simulink model "SCM_PD_PENDULUM_OKE"  (R2017b)
settings: Solver=FixedStepAuto  StartTime=0.0  StopTime=40  FixedStep=0.01  RelTol=1e-3
settings Model: Creator=DELL  LastModifiedBy=DELL

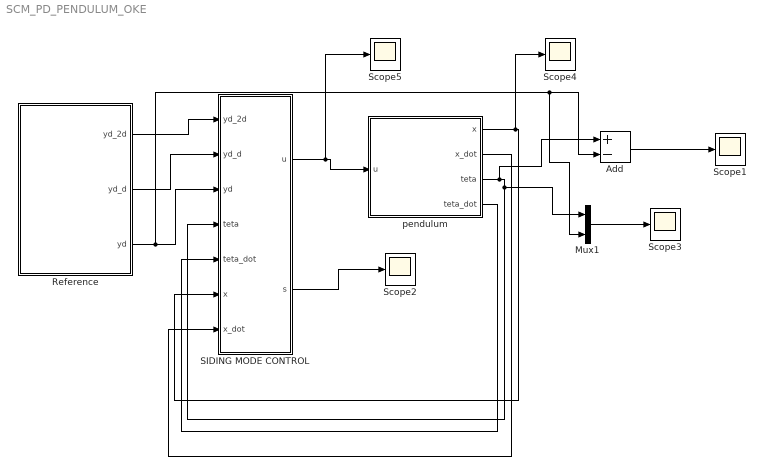
== system SCM_PD_PENDULUM_OKE ==
  Add : Sum  Inputs=+-
  Mux1 : Mux  Inputs=2
  Reference : Subsystem
  "SIDING MODE CONTROL " : MATLAB Function  TreatAsAtomicUnit=on
  Scope{1..5} (5 alike) : Scope
  pendulum : Subsystem
  wires:
  Add/1 -> Scope1/1
  Reference/1(yd_2d) -> "SIDING MODE CONTROL "/1(yd_2d)
  Reference/2(yd_d) -> "SIDING MODE CONTROL "/2(yd_d)
  Reference/3(yd) -> Mux1/2, Add/2, "SIDING MODE CONTROL "/3(yd)
  pendulum/3(teta) -> Add/1, Mux1/1, "SIDING MODE CONTROL "/4(teta)
  pendulum/4(teta_dot) -> "SIDING MODE CONTROL "/5(teta_dot)
  pendulum/1(x) -> Scope4/1, "SIDING MODE CONTROL "/6(x)
  pendulum/2(x_dot) -> "SIDING MODE CONTROL "/7(x_dot)
  Mux1/1 -> Scope3/1
  "SIDING MODE CONTROL "/1(u) -> Scope5/1, pendulum/1(u)
  "SIDING MODE CONTROL "/2(s) -> Scope2/1

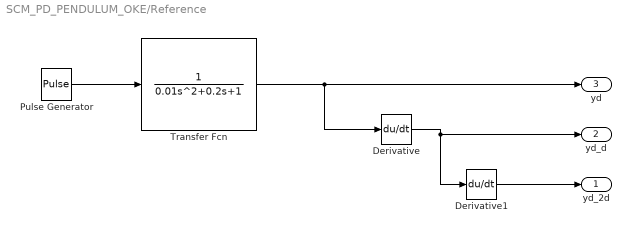
== system SCM_PD_PENDULUM_OKE/Reference ==
  Derivative : Derivative
  Derivative1 : Derivative
  Pulse Generator : DiscretePulseGenerator  PulseType=Time based  Amplitude=pi/3  Period=20  PulseWidth=50
  Transfer Fcn : TransferFcn  Denominator=[0.01 0.2 1]
  yd_2d : Outport  VectorParamsAs1DForOutWhenUnconnected=on
  yd_d : Outport  Port=2  VectorParamsAs1DForOutWhenUnconnected=on
  yd : Outport  Port=3  VectorParamsAs1DForOutWhenUnconnected=on
  wires:
  Transfer Fcn/1 -> Derivative/1, yd/1
  Pulse Generator/1 -> Transfer Fcn/1
  Derivative/1 -> Derivative1/1, yd_d/1
  Derivative1/1 -> yd_2d/1

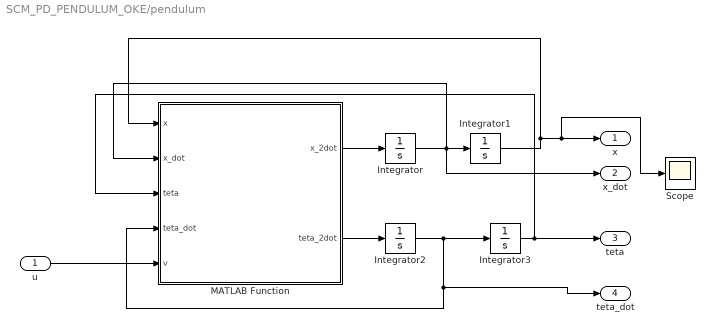
== system SCM_PD_PENDULUM_OKE/pendulum ==
  u : Inport
  Integrator : Integrator
  Integrator1 : Integrator  InitialCondition=0.05
  Integrator2 : Integrator
  Integrator3 : Integrator  InitialCondition=0.05
  MATLAB Function : MATLAB Function  TreatAsAtomicUnit=on
  Scope : Scope
  x : Outport
  x_dot : Outport  Port=2
  teta : Outport  Port=3
  teta_dot : Outport  Port=4
  wires:
  Integrator2/1 -> teta_dot/1, MATLAB Function/4(teta_dot), Integrator3/1
  MATLAB Function/2(teta_2dot) -> Integrator2/1
  Integrator1/1 -> x/1, Scope/1, MATLAB Function/1(x)
  MATLAB Function/1(x_2dot) -> Integrator/1
  Integrator3/1 -> teta/1, MATLAB Function/3(teta)
  Integrator/1 -> x_dot/1, MATLAB Function/2(x_dot), Integrator1/1
  u/1 -> MATLAB Function/5(v)

== matlab function SCM_PD_PENDULUM_OKE/pendulum/MATLAB Function ==
  data: x input; x_2dot output; x_dot input; teta input; teta_dot input; v input; teta_2dot output
function [x_2dot,teta_2dot] = fcn(x,x_dot,teta,teta_dot,v)
global v1 v2
g=9.81; %Gravity(m/s^2)
r=0.051; %Radius of wheel(m)
Mw=0.03; %Mass of wheel(kg)
Mp=1.13; %Mass of body(kg)
Iw=0.000039; %Inertia of the wheel(kg*m^2)
Ip=0.0041; %Inertia of the body(kg*m^2)
L=0.07; %Length to the body's center of mass(m)

%Motor's variables
Km=0.006123; %Motor torque constant(Nm/A)
Ke=0.006087; %Back EMF constant(Vs/rad)
R=3; %Nominal terminal resistance(Ohm)
a1=Mp*L/(Ip+Mp*L^2);
a2=Km*Ke/(R*r*(Ip+Mp*L^2));
a3=Km/(R*(Ip+Mp*L^2));
a4=Mp*g*L/(Ip+Mp*L^2);
b1=2*Km/(R*r*(2*Mw+2*(Iw/r^2)+Mp));
b2=2*Km*Ke/(R*r^2*(2*Mw+2*(Iw/r^2)+Mp));
b3=Mp*L/(2*Mw+2*(Iw/r^2)+Mp);
K=1.0e+03 *[-0.0316   -0.0361    1.6415    0.1272];


teta_2dot = -(a4*teta - 2*a3*v + 2*a2*x + a1*b1*v - a1*b2*x_dot)/(a1*b3 - 1);
x_2dot=-(b1*v - b2*x_dot + a4*b3*teta - 2*a3*b3*v + 2*a2*b3*x)/(a1*b3 - 1);

== matlab function SCM_PD_PENDULUM_OKE/SIDING MODE CONTROL  ==
  data: yd_2d input; u output; yd_d input; yd input; teta input; teta_dot input; s output; x input; x_dot input
function [u,s]= SMC(yd_2d,yd_d,yd,teta,teta_dot,x,x_dot)

g=9.81; %Gravity(m/s^2)
r=0.051; %Radius of wheel(m)
Mw=0.03; %Mass of wheel(kg)
Mp=1.13; %Mass of body(kg)
Iw=0.000039; %Inertia of the wheel(kg*m^2)
Ip=0.0041; %Inertia of the body(kg*m^2)
L=0.07; %Length to the body's center of mass(m)

%Motor's variables
Km=0.006123; %Motor torque constant(Nm/A)
Ke=0.006087; %Back EMF constant(Vs/rad)
R=3; %Nominal terminal resistance(Ohm)
a1=Mp*L/(Ip+Mp*L^2);
a2=Km*Ke/(R*r*(Ip+Mp*L^2));
a3=Km/(R*(Ip+Mp*L^2));
a4=Mp*g*L/(Ip+Mp*L^2);
b1=2*Km/(R*r*(2*Mw+2*(Iw/r^2)+Mp));
b2=2*Km*Ke/(R*r^2*(2*Mw+2*(Iw/r^2)+Mp));
b3=Mp*L/(2*Mw+2*(Iw/r^2)+Mp);

landa=10;k1=20;k=2;%landa=10;k1=20;k=2;
%landa=10;n=2;k=20;
g1=-(a1*b1- 2*a3)/(a1*b3 - 1);
f1=-(a4*teta + 2*a2*x  - a1*b2*x_dot)/(a1*b3 - 1);
g2=-(b1- 2*a3*b3)/(a1*b3 - 1);
f2=-(- b2*x_dot + a4*b3*teta + 2*a2*b3*x)/(a1*b3 - 1);

e1=teta-yd;
e2=x-yd;
e1_d=teta_dot-yd_d;
e2_d=x_dot-yd_d;
s1=e1_d+landa*e1;
s2=e2_d+landa*e2;
s=s1;
u2=1/g2*(yd_2d-landa*e2_d-f2-k1*s2-k*sign(s2));
 u1=1/g1*(yd_2d-landa*e1_d-f1-k1*s1-k*sign(s1));
 u=u1;
%u2=1/g2*(yd_2d-landa*e2_d-f2-k1*s2-k*sign(s2));
%u1=1/g1*(yd_2d-landa*e1_d-f1-k1*s1-k*sign(s1));
